simulink model "GIT_Shared_Model_Example"  (R2019b)
settings: Solver=FixedStepDiscrete  StartTime=0.0  StopTime=10  FixedStep=0.01  RelTol=1e-3  EnableMultiTasking=on
InitFcn:
  | clear mex;
undefined symbols (not defined in the file): asbcbaseini_C, ibatini_C, k_icalpl_C, scsocini_C, stopengstmode_C, t_bmaxini_C, t_bminini_C, t_vminddstr_C, TSB_Coulomb_float, TSB_Dc_float, TSB_Pwr_float, TSB_R_float, TSB_Soc, TSB_Tbatt, TSB_Tbatt_float, TSB_value_float, TSB_Volt_float, v_bcini_C, v_bcmaxini_C
libraries: Utility_Block_Library x22, AMO_Block_Library x2
(part 5 of 5)

== system GIT_Shared_Model_Example/Simulink Function/Model Header ==

== system GIT_Shared_Model_Example/Simulink Function/Model Source ==

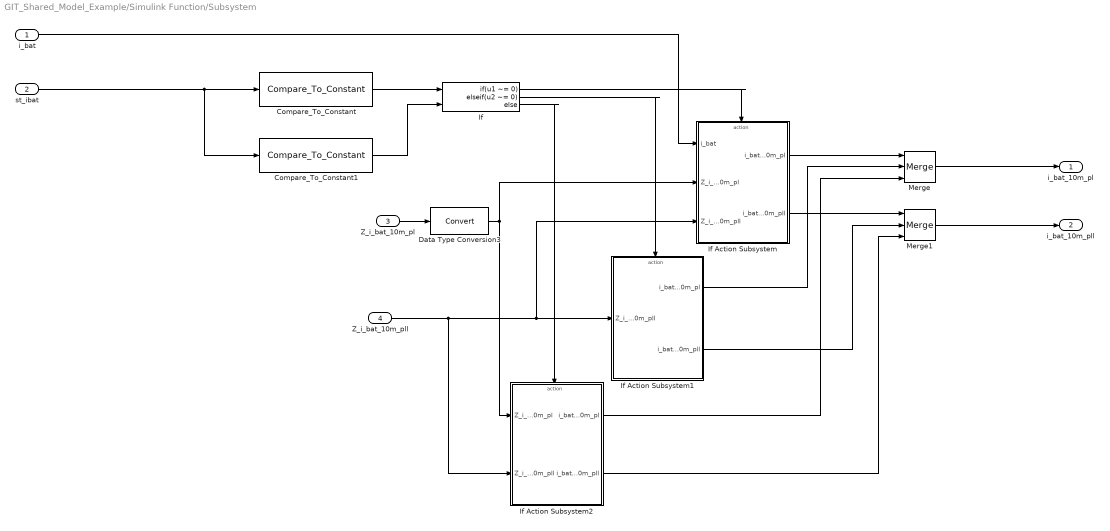
== system GIT_Shared_Model_Example/Simulink Function/Subsystem ==
  i_bat : Inport  Tag=#AMO_Lib
      settings: AttributesFormatString=%<Tag>\n%<Description>\nSampleTime = %<SampleTime>
  st_ibat : Inport  Tag=#AMO_Lib  Port=2
      settings: AttributesFormatString=%<Tag>\n%<Description>\nSampleTime = %<SampleTime>
  Z_i_bat_10m_pl : Inport  Tag=#AMO_Lib  Port=3
      settings: AttributesFormatString=%<Tag>\n%<Description>\nSampleTime = %<SampleTime>
  Z_i_bat_10m_pll : Inport  Tag=#AMO_Lib  Port=4
      settings: AttributesFormatString=%<Tag>\n%<Description>\nSampleTime = %<SampleTime>
  Compare_To_Constant : AMO_Block_Library/AMO_Original_Blocks/CompareTo/Compare_To_Constant  Tag=#AMO_Lib  relop===  const=1  OutDataTypeStr_constant=Inherit: Inherit via back propagation
      settings: SourceProductName=AMO_Block_Library
      settings: AttributesFormatString=|
      | %<Tag>
      | 比較定数のデータ型： %<OutDataTypeStr_constant>
  Compare_To_Constant1 : AMO_Block_Library/AMO_Original_Blocks/CompareTo/Compare_To_Constant  Tag=#AMO_Lib  relop===  const=0  OutDataTypeStr_constant=Inherit: Inherit via back propagation
      settings: SourceProductName=AMO_Block_Library
      settings: AttributesFormatString=|
      | %<Tag>
      | 比較定数のデータ型： %<OutDataTypeStr_constant>
  Data Type Conversion3 : DataTypeConversion  Tag=#AMO_Lib  OutMin=OutMin  OutMax=OutMax  ConvertRealWorld=Stored Integer (SI)  SampleTime=SampleTime  SaturateOnIntegerOverflow=on  RndMeth=Zero  mask{OutMin=[], OutMax=[], OutDataTypeStr=Inherit: Inherit via back propagation, LockScale=off, ConvertRealWorld=Stored Integer (SI), RndMeth=Zero, SaturateOnIntegerOverflow=on, SampleTime=-1}
      mask prompts: OutMin "Simulink:blkprm_prompts:OutputDesignMin"; OutMax "Simulink:blkprm_prompts:OutputDesignMax"; OutDataTypeStr "Simulink:blkprm_prompts:OUTPUT_UNIFIEDDATATYPE"; LockScale "Simulink:blkprm_prompts:LockScale"; ConvertRealWorld "Simulink:blkprm_prompts:DtypeCnvInputOutputValue"; RndMeth "Simulink:blkprm_prompts:SPP_RndMeth_ID"; SaturateOnIntegerOverflow "Simulink:blkprm_prompts:AllBlksSaturate"; SampleTime "Simulink:blkprm_prompts:AllBlksSampleTime"
      mask help:
      | 入力を出力のデータ型とスケーリングに変換します。
      |
      | この変換には 2 つの目的があります。1 つは入力と出力の実際値を等しくすることです。もう 1 つは入力と出力の整数格納値を等しくすることです。オーバーフローと量子化誤差があると、この目的を完全に達成することができません。
      settings: AttributesFormatString=%<Tag>\nOutDataType = %<OutDataTypeStr>
      mask TypeOptions OutMin: OutMin
      mask TypeOptions OutMax: OutMax
      mask TypeOptions OutDataTypeStr: OutDataTypeStr
      mask TypeOptions LockScale: LockScale
      mask TypeOptions ConvertRealWorld: ConvertRealWorld
      mask TypeOptions RndMeth: RndMeth
      mask TypeOptions SaturateOnIntegerOverflow: SaturateOnIntegerOverflow
      mask TypeOptions SampleTime: SampleTime
      mask DialogControl OutMin Prompt: 出力の最小値:
      mask DialogControl OutMax Prompt: 出力の最大値:
      mask DialogControl OutDataTypeStr Prompt: 出力データ型:
      mask DialogControl LockScale Prompt: 固定小数点ツールによる変更に対して出力データ型の設定をロックする
      mask DialogControl ConvertRealWorld Prompt: 等価な値をもつ入力と出力:
      mask DialogControl RndMeth Prompt: 整数丸めモード:
      mask DialogControl SaturateOnIntegerOverflow Prompt: 整数オーバーフローで飽和
      mask DialogControl SampleTime Prompt: サンプル時間 (継承は -1):
  If : If  Tag=#AMO_Lib  NumInputs=2  IfExpression=u1 ~= 0  ElseIfExpressions=u2 ~= 0
      settings: AttributesFormatString=%<Tag>
  If Action Subsystem : Subsystem  TreatAsAtomicUnit=on
      settings: AttributesFormatString=SampleTime = %<SystemSampleTime>
  If Action Subsystem1 : Subsystem  TreatAsAtomicUnit=on
      settings: AttributesFormatString=SampleTime = %<SystemSampleTime>
  If Action Subsystem2 : Subsystem  TreatAsAtomicUnit=on
      settings: AttributesFormatString=SampleTime = %<SystemSampleTime>
  Merge : Merge  Tag=#AMO_Lib  Inputs=3  InitialOutput=0
      settings: AttributesFormatString=%<Tag>\nInitialOutput = %<InitialOutput>
  Merge1 : Merge  Tag=#AMO_Lib  Inputs=3  InitialOutput=0
      settings: AttributesFormatString=%<Tag>\nInitialOutput = %<InitialOutput>
  i_bat_10m_pl : Outport  Tag=#AMO_Lib
      settings: AttributesFormatString=%<Tag>\n%<Description>\nInitialOutput = %<InitialOutput>
  i_bat_10m_pll : Outport  Tag=#AMO_Lib  Port=2
      settings: AttributesFormatString=%<Tag>\n%<Description>\nInitialOutput = %<InitialOutput>
  wires:
  Compare_To_Constant/1 -> If/1
  If Action Subsystem2/1(i_bat_10m_pl) -> Merge/3
  Compare_To_Constant1/1 -> If/2
  If/3 -> If Action Subsystem2/Action
  Z_i_bat_10m_pl/1 -> Data Type Conversion3/1
  If/2 -> If Action Subsystem1/Action
  If Action Subsystem1/1(i_bat_10m_pl) -> Merge/2
  st_ibat/1 -> Compare_To_Constant/1, Compare_To_Constant1/1
  If Action Subsystem/1(i_bat_10m_pl) -> Merge/1
  If Action Subsystem/2(i_bat_10m_pll) -> Merge1/1
  If Action Subsystem1/2(i_bat_10m_pll) -> Merge1/2
  If Action Subsystem2/2(i_bat_10m_pll) -> Merge1/3
  If/1 -> If Action Subsystem/Action
  i_bat/1 -> If Action Subsystem/1(i_bat)
  Z_i_bat_10m_pll/1 -> If Action Subsystem/3(Z_i_bat_10m_pll), If Action Subsystem1/1(Z_i_bat_10m_pll), If Action Subsystem2/2(Z_i_bat_10m_pll)
  Merge/1 -> i_bat_10m_pl/1
  Merge1/1 -> i_bat_10m_pll/1
  Data Type Conversion3/1 -> If Action Subsystem/2(Z_i_bat_10m_pl), If Action Subsystem2/1(Z_i_bat_10m_pl)

== system GIT_Shared_Model_Example/Simulink Function/System Outputs ==

== system GIT_Shared_Model_Example/Simulink Function/System Update ==

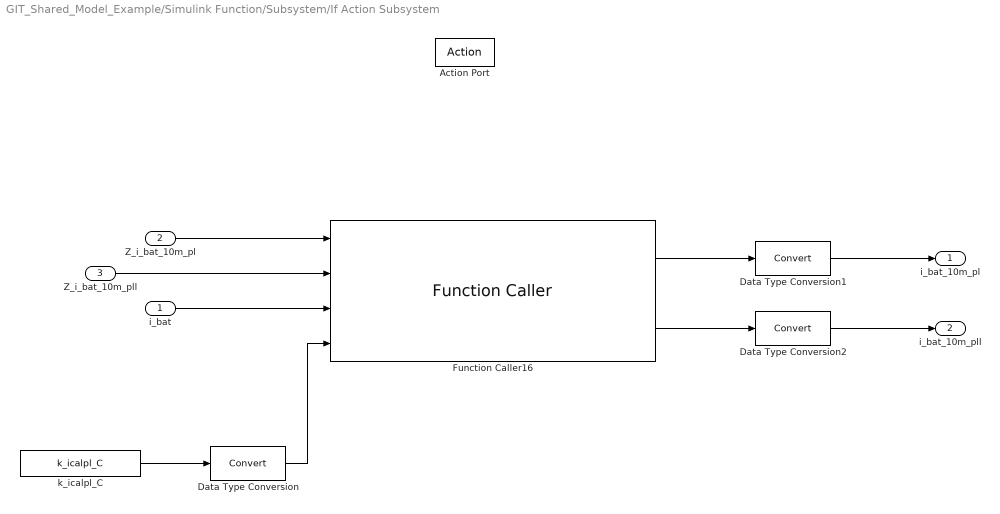
== system GIT_Shared_Model_Example/Simulink Function/Subsystem/If Action Subsystem ==
  i_bat : Inport  Tag=#AMO_Lib
      settings: AttributesFormatString=%<Tag>\n%<Description>\nSampleTime = %<SampleTime>
  Z_i_bat_10m_pl : Inport  Tag=#AMO_Lib  Port=2
      settings: AttributesFormatString=%<Tag>\n%<Description>\nSampleTime = %<SampleTime>
  Z_i_bat_10m_pll : Inport  Tag=#AMO_Lib  Port=3
      settings: AttributesFormatString=%<Tag>\n%<Description>\nSampleTime = %<SampleTime>
  Action Port : ActionPort  Tag=#AMO_Lib  ActionPortLabel=if(u1 ~= 0)
      settings: AttributesFormatString=%<Tag>\nInitializeStates = %<InitializeStates>
  Data Type Conversion : DataTypeConversion  Tag=#AMO_Lib  OutMin=OutMin  OutMax=OutMax  ConvertRealWorld=Stored Integer (SI)  SampleTime=SampleTime  SaturateOnIntegerOverflow=on  RndMeth=Zero  mask{OutMin=[], OutMax=[], OutDataTypeStr=Inherit: Inherit via back propagation, LockScale=off, ConvertRealWorld=Stored Integer (SI), RndMeth=Zero, SaturateOnIntegerOverflow=on, SampleTime=-1}
      mask prompts: OutMin "Simulink:blkprm_prompts:OutputDesignMin"; OutMax "Simulink:blkprm_prompts:OutputDesignMax"; OutDataTypeStr "Simulink:blkprm_prompts:OUTPUT_UNIFIEDDATATYPE"; LockScale "Simulink:blkprm_prompts:LockScale"; ConvertRealWorld "Simulink:blkprm_prompts:DtypeCnvInputOutputValue"; RndMeth "Simulink:blkprm_prompts:SPP_RndMeth_ID"; SaturateOnIntegerOverflow "Simulink:blkprm_prompts:AllBlksSaturate"; SampleTime "Simulink:blkprm_prompts:AllBlksSampleTime"
      mask help:
      | 入力を出力のデータ型とスケーリングに変換します。
      |
      | この変換には 2 つの目的があります。1 つは入力と出力の実際値を等しくすることです。もう 1 つは入力と出力の整数格納値を等しくすることです。オーバーフローと量子化誤差があると、この目的を完全に達成することができません。
      settings: AttributesFormatString=%<Tag>\nOutDataType = %<OutDataTypeStr>
      mask TypeOptions OutMin: OutMin
      mask TypeOptions OutMax: OutMax
      mask TypeOptions OutDataTypeStr: OutDataTypeStr
      mask TypeOptions LockScale: LockScale
      mask TypeOptions ConvertRealWorld: ConvertRealWorld
      mask TypeOptions RndMeth: RndMeth
      mask TypeOptions SaturateOnIntegerOverflow: SaturateOnIntegerOverflow
      mask TypeOptions SampleTime: SampleTime
      mask DialogControl OutMin Prompt: 出力の最小値:
      mask DialogControl OutMax Prompt: 出力の最大値:
      mask DialogControl OutDataTypeStr Prompt: 出力データ型:
      mask DialogControl LockScale Prompt: 固定小数点ツールによる変更に対して出力データ型の設定をロックする
      mask DialogControl ConvertRealWorld Prompt: 等価な値をもつ入力と出力:
      mask DialogControl RndMeth Prompt: 整数丸めモード:
      mask DialogControl SaturateOnIntegerOverflow Prompt: 整数オーバーフローで飽和
      mask DialogControl SampleTime Prompt: サンプル時間 (継承は -1):
  Data Type Conversion1 : DataTypeConversion  Tag=#AMO_Lib  OutMin=OutMin  OutMax=OutMax  ConvertRealWorld=Stored Integer (SI)  SampleTime=SampleTime  SaturateOnIntegerOverflow=on  RndMeth=Zero  mask{OutMin=[], OutMax=[], OutDataTypeStr=Inherit: Inherit via back propagation, LockScale=off, ConvertRealWorld=Stored Integer (SI), RndMeth=Zero, SaturateOnIntegerOverflow=on, SampleTime=-1}
      mask prompts: OutMin "Simulink:blkprm_prompts:OutputDesignMin"; OutMax "Simulink:blkprm_prompts:OutputDesignMax"; OutDataTypeStr "Simulink:blkprm_prompts:OUTPUT_UNIFIEDDATATYPE"; LockScale "Simulink:blkprm_prompts:LockScale"; ConvertRealWorld "Simulink:blkprm_prompts:DtypeCnvInputOutputValue"; RndMeth "Simulink:blkprm_prompts:SPP_RndMeth_ID"; SaturateOnIntegerOverflow "Simulink:blkprm_prompts:AllBlksSaturate"; SampleTime "Simulink:blkprm_prompts:AllBlksSampleTime"
      mask help:
      | 入力を出力のデータ型とスケーリングに変換します。
      |
      | この変換には 2 つの目的があります。1 つは入力と出力の実際値を等しくすることです。もう 1 つは入力と出力の整数格納値を等しくすることです。オーバーフローと量子化誤差があると、この目的を完全に達成することができません。
      settings: AttributesFormatString=%<Tag>\nOutDataType = %<OutDataTypeStr>
      mask TypeOptions OutMin: OutMin
      mask TypeOptions OutMax: OutMax
      mask TypeOptions OutDataTypeStr: OutDataTypeStr
      mask TypeOptions LockScale: LockScale
      mask TypeOptions ConvertRealWorld: ConvertRealWorld
      mask TypeOptions RndMeth: RndMeth
      mask TypeOptions SaturateOnIntegerOverflow: SaturateOnIntegerOverflow
      mask TypeOptions SampleTime: SampleTime
      mask DialogControl OutMin Prompt: 出力の最小値:
      mask DialogControl OutMax Prompt: 出力の最大値:
      mask DialogControl OutDataTypeStr Prompt: 出力データ型:
      mask DialogControl LockScale Prompt: 固定小数点ツールによる変更に対して出力データ型の設定をロックする
      mask DialogControl ConvertRealWorld Prompt: 等価な値をもつ入力と出力:
      mask DialogControl RndMeth Prompt: 整数丸めモード:
      mask DialogControl SaturateOnIntegerOverflow Prompt: 整数オーバーフローで飽和
      mask DialogControl SampleTime Prompt: サンプル時間 (継承は -1):
  Data Type Conversion2 : DataTypeConversion  Tag=#AMO_Lib  OutMin=OutMin  OutMax=OutMax  ConvertRealWorld=Stored Integer (SI)  SampleTime=SampleTime  SaturateOnIntegerOverflow=on  RndMeth=Zero  mask{OutMin=[], OutMax=[], OutDataTypeStr=Inherit: Inherit via back propagation, LockScale=off, ConvertRealWorld=Stored Integer (SI), RndMeth=Zero, SaturateOnIntegerOverflow=on, SampleTime=-1}
      mask prompts: OutMin "Simulink:blkprm_prompts:OutputDesignMin"; OutMax "Simulink:blkprm_prompts:OutputDesignMax"; OutDataTypeStr "Simulink:blkprm_prompts:OUTPUT_UNIFIEDDATATYPE"; LockScale "Simulink:blkprm_prompts:LockScale"; ConvertRealWorld "Simulink:blkprm_prompts:DtypeCnvInputOutputValue"; RndMeth "Simulink:blkprm_prompts:SPP_RndMeth_ID"; SaturateOnIntegerOverflow "Simulink:blkprm_prompts:AllBlksSaturate"; SampleTime "Simulink:blkprm_prompts:AllBlksSampleTime"
      mask help:
      | 入力を出力のデータ型とスケーリングに変換します。
      |
      | この変換には 2 つの目的があります。1 つは入力と出力の実際値を等しくすることです。もう 1 つは入力と出力の整数格納値を等しくすることです。オーバーフローと量子化誤差があると、この目的を完全に達成することができません。
      settings: AttributesFormatString=%<Tag>\nOutDataType = %<OutDataTypeStr>
      mask TypeOptions OutMin: OutMin
      mask TypeOptions OutMax: OutMax
      mask TypeOptions OutDataTypeStr: OutDataTypeStr
      mask TypeOptions LockScale: LockScale
      mask TypeOptions ConvertRealWorld: ConvertRealWorld
      mask TypeOptions RndMeth: RndMeth
      mask TypeOptions SaturateOnIntegerOverflow: SaturateOnIntegerOverflow
      mask TypeOptions SampleTime: SampleTime
      mask DialogControl OutMin Prompt: 出力の最小値:
      mask DialogControl OutMax Prompt: 出力の最大値:
      mask DialogControl OutDataTypeStr Prompt: 出力データ型:
      mask DialogControl LockScale Prompt: 固定小数点ツールによる変更に対して出力データ型の設定をロックする
      mask DialogControl ConvertRealWorld Prompt: 等価な値をもつ入力と出力:
      mask DialogControl RndMeth Prompt: 整数丸めモード:
      mask DialogControl SaturateOnIntegerOverflow Prompt: 整数オーバーフローで飽和
      mask DialogControl SampleTime Prompt: サンプル時間 (継承は -1):
  Function Caller16 : FunctionCaller  FunctionPrototype=[S15_refout3,S31_refls] = GE_Cal_ref4s(S15_refhs,S31_refls,S15_obj3,U16_cref)  InputArgumentSpecifications=int16(1),int32(1),int16(1),uint16(1)  OutputArgumentSpecifications=int16(1),int32(1)
  k_icalpl_C : Constant  Tag=#AMO_Lib  Value=k_icalpl_C
      settings: AttributesFormatString=%<Tag>\nOutDataType = %<OutDataTypeStr>
  i_bat_10m_pl : Outport  Tag=#AMO_Lib
      settings: AttributesFormatString=%<Tag>\n%<Description>\nInitialOutput = %<InitialOutput>
  i_bat_10m_pll : Outport  Tag=#AMO_Lib  Port=2
      settings: AttributesFormatString=%<Tag>\n%<Description>\nInitialOutput = %<InitialOutput>
  wires:
  i_bat/1 -> Function Caller16/3
  Function Caller16/1 -> Data Type Conversion1/1
  Function Caller16/2 -> Data Type Conversion2/1
  Z_i_bat_10m_pll/1 -> Function Caller16/2
  k_icalpl_C/1 -> Data Type Conversion/1
  Data Type Conversion/1 -> Function Caller16/4
  Data Type Conversion1/1 -> i_bat_10m_pl/1
  Data Type Conversion2/1 -> i_bat_10m_pll/1
  Z_i_bat_10m_pl/1 -> Function Caller16/1

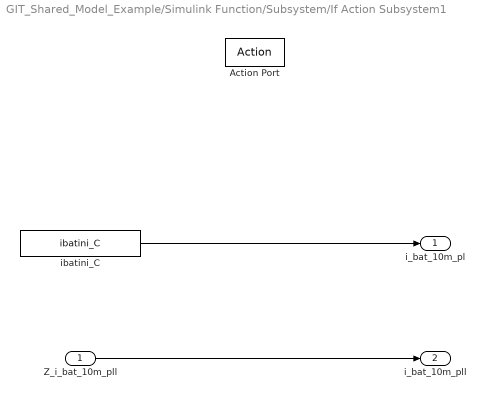
== system GIT_Shared_Model_Example/Simulink Function/Subsystem/If Action Subsystem1 ==
  Z_i_bat_10m_pll : Inport  Tag=#AMO_Lib
      settings: AttributesFormatString=%<Tag>\n%<Description>\nSampleTime = %<SampleTime>
  Action Port : ActionPort  Tag=#AMO_Lib  ActionPortLabel=elseif(u2 ~= 0)
      settings: AttributesFormatString=%<Tag>\nInitializeStates = %<InitializeStates>
  ibatini_C : Constant  Tag=#AMO_Lib  Value=ibatini_C
      settings: AttributesFormatString=%<Tag>\nOutDataType = %<OutDataTypeStr>
  i_bat_10m_pl : Outport  Tag=#AMO_Lib
      settings: AttributesFormatString=%<Tag>\n%<Description>\nInitialOutput = %<InitialOutput>
  i_bat_10m_pll : Outport  Tag=#AMO_Lib  Port=2
      settings: AttributesFormatString=%<Tag>\n%<Description>\nInitialOutput = %<InitialOutput>
  wires:
  ibatini_C/1 -> i_bat_10m_pl/1
  Z_i_bat_10m_pll/1 -> i_bat_10m_pll/1

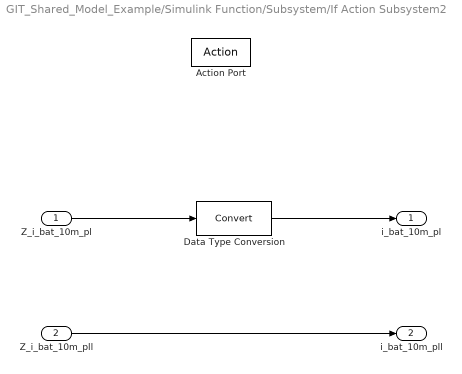
== system GIT_Shared_Model_Example/Simulink Function/Subsystem/If Action Subsystem2 ==
  Z_i_bat_10m_pl : Inport  Tag=#AMO_Lib
      settings: AttributesFormatString=%<Tag>\n%<Description>\nSampleTime = %<SampleTime>
  Z_i_bat_10m_pll : Inport  Tag=#AMO_Lib  Port=2
      settings: AttributesFormatString=%<Tag>\n%<Description>\nSampleTime = %<SampleTime>
  Action Port : ActionPort  Tag=#AMO_Lib  ActionPortLabel=else
      settings: AttributesFormatString=%<Tag>\nInitializeStates = %<InitializeStates>
  Data Type Conversion : DataTypeConversion  Tag=#AMO_Lib  OutMin=OutMin  OutMax=OutMax  ConvertRealWorld=Stored Integer (SI)  SampleTime=SampleTime  SaturateOnIntegerOverflow=on  RndMeth=Zero  mask{OutMin=[], OutMax=[], OutDataTypeStr=Inherit: Inherit via back propagation, LockScale=off, ConvertRealWorld=Stored Integer (SI), RndMeth=Zero, SaturateOnIntegerOverflow=on, SampleTime=-1}
      mask prompts: OutMin "Simulink:blkprm_prompts:OutputDesignMin"; OutMax "Simulink:blkprm_prompts:OutputDesignMax"; OutDataTypeStr "Simulink:blkprm_prompts:OUTPUT_UNIFIEDDATATYPE"; LockScale "Simulink:blkprm_prompts:LockScale"; ConvertRealWorld "Simulink:blkprm_prompts:DtypeCnvInputOutputValue"; RndMeth "Simulink:blkprm_prompts:SPP_RndMeth_ID"; SaturateOnIntegerOverflow "Simulink:blkprm_prompts:AllBlksSaturate"; SampleTime "Simulink:blkprm_prompts:AllBlksSampleTime"
      mask help:
      | 入力を出力のデータ型とスケーリングに変換します。
      |
      | この変換には 2 つの目的があります。1 つは入力と出力の実際値を等しくすることです。もう 1 つは入力と出力の整数格納値を等しくすることです。オーバーフローと量子化誤差があると、この目的を完全に達成することができません。
      settings: AttributesFormatString=%<Tag>\nOutDataType = %<OutDataTypeStr>
      mask TypeOptions OutMin: OutMin
      mask TypeOptions OutMax: OutMax
      mask TypeOptions OutDataTypeStr: OutDataTypeStr
      mask TypeOptions LockScale: LockScale
      mask TypeOptions ConvertRealWorld: ConvertRealWorld
      mask TypeOptions RndMeth: RndMeth
      mask TypeOptions SaturateOnIntegerOverflow: SaturateOnIntegerOverflow
      mask TypeOptions SampleTime: SampleTime
      mask DialogControl OutMin Prompt: 出力の最小値:
      mask DialogControl OutMax Prompt: 出力の最大値:
      mask DialogControl OutDataTypeStr Prompt: 出力データ型:
      mask DialogControl LockScale Prompt: 固定小数点ツールによる変更に対して出力データ型の設定をロックする
      mask DialogControl ConvertRealWorld Prompt: 等価な値をもつ入力と出力:
      mask DialogControl RndMeth Prompt: 整数丸めモード:
      mask DialogControl SaturateOnIntegerOverflow Prompt: 整数オーバーフローで飽和
      mask DialogControl SampleTime Prompt: サンプル時間 (継承は -1):
  i_bat_10m_pl : Outport  Tag=#AMO_Lib
      settings: AttributesFormatString=%<Tag>\n%<Description>\nInitialOutput = %<InitialOutput>
  i_bat_10m_pll : Outport  Tag=#AMO_Lib  Port=2
      settings: AttributesFormatString=%<Tag>\n%<Description>\nInitialOutput = %<InitialOutput>
  wires:
  Z_i_bat_10m_pl/1 -> Data Type Conversion/1
  Z_i_bat_10m_pll/1 -> i_bat_10m_pll/1
  Data Type Conversion/1 -> i_bat_10m_pl/1
